simulink model "ComfortMdRStEnCtrl"  (R2018b)
settings: Solver=FixedStepDiscrete  StartTime=0.0  StopTime=10.0  FixedStep=0.01  RelTol=1e-3
undefined symbols (not defined in the file or in its folder): data, KeSMSw4SSecRwLtStLgrstOtwdInwdClosePos1_Val, KeSMSw4SSecRwLtStLgrstUpwdDnwdClosePos1_Val, KeSMSw4SSecRwLtStLgrstUpwdDnwdClosePos2_Val, KeSMSw4SSecRwRtStLgrstUpwdDnwdOpenPos1_Val, SecRwRtStBkRclnEn_Clear, SecRwRtStBkRclnEn_Set, SecRwRtStLgrstInwdOtwdEn_Clear, SecRwRtStLgrstInwdOtwdEn_Set, SecRwRtStLgrstUpwdDnwdEn_Clear, SecRwRtStLgrstUpwdDnwdEn_Set, ZeroREn_Clear, ZeroREn_Set
libraries: simulink x1
settings Model: Creator=sn2xws  LastModifiedBy=sn2xws
settings Model: ModifiedHistory=|
  | 2024.6.19 V1.1.0 模式流程V1.6
  | 2025.4.18 V1.10.0 腿托收流程中标定使用错误问题修复
settings DataIOCC: SaveFormat=StructureWithTime
settings OptimizationCC: DefaultParameterBehavior=Inlined  EnhancedBackFolding=on  PassReuseOutputArgsAs=Individual arguments  ZeroExternalMemoryAtStartup=off  ZeroInternalMemoryAtStartup=off  OptimizeBlockOrder=speed  DifferentSizesBufferReuse=on  OptimizationCustomize=off
settings DebuggingCC: ParameterTunabilityLossMsg=error
settings SFSimCC: MATLABDynamicMemAlloc=off
settings RTWCC: SystemTargetFile=autosar.tlc  GenCodeOnly=on  TemplateMakefile=ert_default_tmf  Description=AUTOSAR  GenerateReport=on  IncludeHyperlinkInReport=on  LaunchReport=on  GenerateTraceInfo=on  GenerateTraceReport=on  GenerateTraceReportSl=on  GenerateTraceReportSf=on  GenerateTraceReportEml=on
settings CodeAppCC: ForceParamTrailComments=on  IgnoreCustomStorageClasses=off  OperatorAnnotations=on  SimulinkDataObjDesc=on  SFDataObjDesc=on  InsertBlockDesc=on
settings STFCustomTargetCC: TargetLangStandard=C99 (ISO)  MultiwordLength=256  ParMdlRefBuildCompliant=on  CompOptLevelCompliant=on  IncludeMdlTerminateFcn=off  CombineOutputUpdateFcns=on  SuppressErrorStatus=on  ERTCustomFileBanners=on  SupportNonFinite=off  SupportComplex=off  SupportContinuousTime=off  SupportNonInlinedSFcns=off  RemoveResetFunc=on  MATLABClassNameForMDSCustomization=Simulink.SoftwareTarget.ERTCustomization  AutosarCompliant=on  UseToolchainInfoCompliant=on  LookupTableObjectStructAxisOrder=2,1,3,4,...  LUTObjectStructOrderEvenSpacing=Size,Table,Breakpoints  SystemTargetFile=autosar.tlc
settings ERTTargetCC: TargetLangStandard=C99 (ISO)  ConcurrentExecutionCompliant=off  IncludeMdlTerminateFcn=off  SuppressErrorStatus=on  SupportNonFinite=off  SupportComplex=off  ModelStepFunctionPrototypeControlCompliant=off  CPPClassGenCompliant=off  AutosarCompliant=on  LookupTableObjectStructAxisOrder=2,1,3,4,...  LUTObjectStructOrderEvenSpacing=Size,Table,Breakpoints  InlinedParameterPlacement=NonHierarchical  ERTCustomFileTemplate=example_file_process.tlc  ERTFilePackagingFormat=Compact

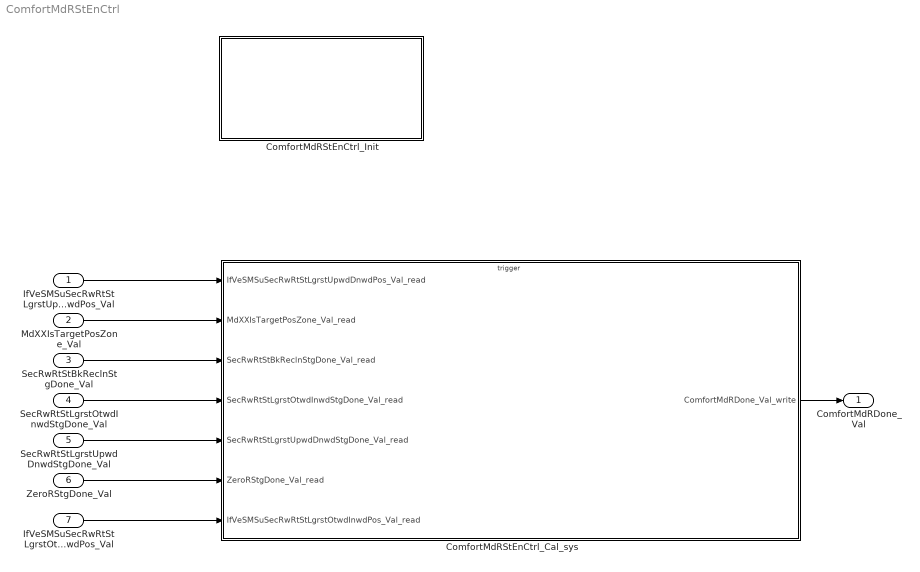
== system ComfortMdRStEnCtrl ==
  IfVeSMSuSecRwRtStLgrstUpwdDnwdPos_Val : Inport  OutDataTypeStr=uint16  PortDimensions=1
  MdXXIsTargetPosZone_Val : Inport  Port=2  OutDataTypeStr=uint32  PortDimensions=1
  SecRwRtStBkReclnStgDone_Val : Inport  Port=3  OutDataTypeStr=boolean  PortDimensions=1
  SecRwRtStLgrstOtwdInwdStgDone_Val : Inport  Port=4  OutDataTypeStr=boolean  PortDimensions=1
  SecRwRtStLgrstUpwdDnwdStgDone_Val : Inport  Port=5  OutDataTypeStr=boolean  PortDimensions=1
  ZeroRStgDone_Val : Inport  Port=6  OutDataTypeStr=boolean  PortDimensions=1
  IfVeSMSuSecRwRtStLgrstOtwdInwdPos_Val : Inport  Port=7  OutDataTypeStr=uint16  PortDimensions=1
  ComfortMdRStEnCtrl_Cal_sys : Subsystem
  ComfortMdRStEnCtrl_Init : Subsystem
  ComfortMdRDone_Val : Outport  OutDataTypeStr=uint8  PortDimensions=1
  wires:
  IfVeSMSuSecRwRtStLgrstUpwdDnwdPos_Val/1 -> ComfortMdRStEnCtrl_Cal_sys/1(IfVeSMSuSecRwRtStLgrstUpwdDnwdPos_Val_read)
  MdXXIsTargetPosZone_Val/1 -> ComfortMdRStEnCtrl_Cal_sys/2(MdXXIsTargetPosZone_Val_read)
  SecRwRtStBkReclnStgDone_Val/1 -> ComfortMdRStEnCtrl_Cal_sys/3(SecRwRtStBkReclnStgDone_Val_read)
  SecRwRtStLgrstOtwdInwdStgDone_Val/1 -> ComfortMdRStEnCtrl_Cal_sys/4(SecRwRtStLgrstOtwdInwdStgDone_Val_read)
  SecRwRtStLgrstUpwdDnwdStgDone_Val/1 -> ComfortMdRStEnCtrl_Cal_sys/5(SecRwRtStLgrstUpwdDnwdStgDone_Val_read)
  ZeroRStgDone_Val/1 -> ComfortMdRStEnCtrl_Cal_sys/6(ZeroRStgDone_Val_read)
  ComfortMdRStEnCtrl_Cal_sys/1(ComfortMdRDone_Val_write) -> ComfortMdRDone_Val/1
  IfVeSMSuSecRwRtStLgrstOtwdInwdPos_Val/1 -> ComfortMdRStEnCtrl_Cal_sys/7(IfVeSMSuSecRwRtStLgrstOtwdInwdPos_Val_read)

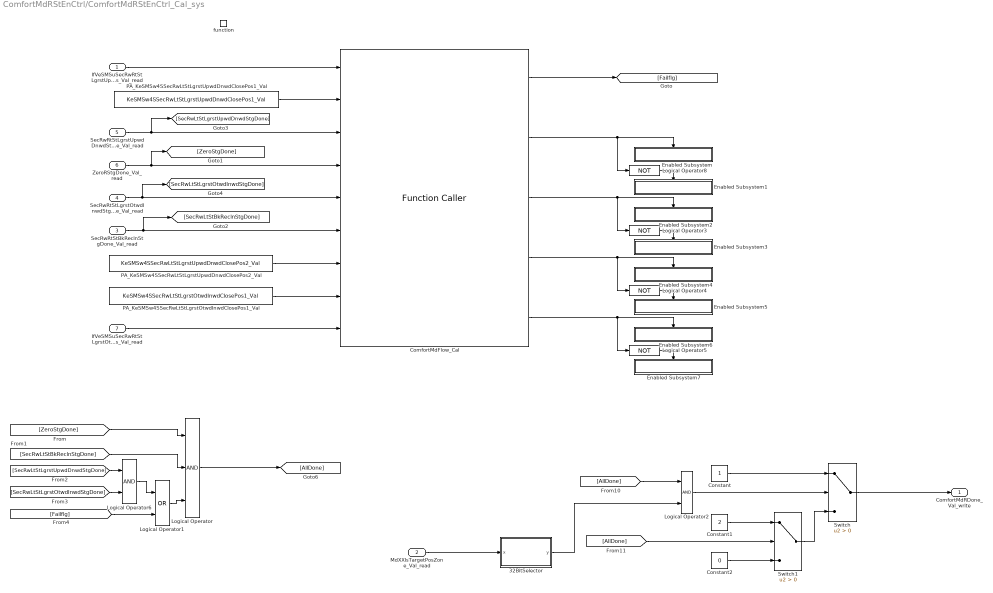
== system ComfortMdRStEnCtrl/ComfortMdRStEnCtrl_Cal_sys ==
  IfVeSMSuSecRwRtStLgrstUpwdDnwdPos_Val_read : Inport
  MdXXIsTargetPosZone_Val_read : Inport  Port=2
  SecRwRtStBkReclnStgDone_Val_read : Inport  Port=3
  SecRwRtStLgrstOtwdInwdStgDone_Val_read : Inport  Port=4
  SecRwRtStLgrstUpwdDnwdStgDone_Val_read : Inport  Port=5
  ZeroRStgDone_Val_read : Inport  Port=6
  IfVeSMSuSecRwRtStLgrstOtwdInwdPos_Val_read : Inport  Port=7
  function : TriggerPort  TriggerType=function-call  IsSimulinkFunction=on  FunctionName=ComfortMdRStEnCtrl_Cal  VariantControl=(inherit)
  32BitSelector : Subsystem  mask(32 Bit Selector){BitNum=12}
      mask prompts: BitNum "Select Bit Number"
      mask help: Allows selection of a particular bit (0-31) out of a packed word up to 32 bits long. Output will be true if the bit number selected via the mask parameter is equal to one.
      mask TypeOptions BitNum: 0 | 1 | 2 | 3 | 4 | 5 | 6 | 7 | 8 | 9 | 10 | 11 | 12 | 13 | 14 | 15 | 16 | 17 | 18 | 19 | 20 | 21 | 22 | 23 | 24 | 25 | 26 | 27 | 28 | 29 | 30 | 31
      mask Display:
      | text(0.5, 0.8,'BIT','horizontalAlignment','center')
      | text(0.5, 0.5,'SELECTOR','horizontalAlignment','center')
      | text(0.5, 0.2,['-- Bit ',char(get_param(gcb,'BitNum')),' --'],'horizontalAlignment','center')
  ComfortMdFlow_Cal : FunctionCaller  FunctionPrototype=[Failflg,LgrstInwdOtwdEn,LgrstUpwdDnwdEn,ZeroEn,BkReclnEn] = ComfortMdFlow_Cal(LgrstUpwdDnwdPos,LgrstUpwdDnwdClosePos1,LgrstUpwdStgDone,ZeroStgDone,LgrstInwdStgDone,BkReclnStgDone,LgrstUpwdDnwdClosePos2,LgrstInwdOtwdClosePos1,LgrstInwdOtwdPos)  InputArgumentSpecifications=uint16(1), uint16(1), boolean(true), boolean(true), boolean(true), boolean(true), uint16(1), uint16(1), uint16(1)  OutputArgumentSpecifications=boolean(true), boolean(true), boolean(true), boolean(true), boolean(true)
  Constant : Constant  OutDataTypeStr=uint8
  Constant1 : Constant  Value=2  OutDataTypeStr=uint8
  Constant2 : Constant  Value=0  OutDataTypeStr=uint8
  Enabled Subsystem : Subsystem  TreatAsAtomicUnit=on
  Enabled Subsystem1 : Subsystem  TreatAsAtomicUnit=on
  Enabled Subsystem2 : Subsystem  TreatAsAtomicUnit=on
  Enabled Subsystem3 : Subsystem  TreatAsAtomicUnit=on
  Enabled Subsystem4 : Subsystem  TreatAsAtomicUnit=on
  Enabled Subsystem5 : Subsystem  TreatAsAtomicUnit=on
  Enabled Subsystem6 : Subsystem  TreatAsAtomicUnit=on
  Enabled Subsystem7 : Subsystem  TreatAsAtomicUnit=on
  Logical Operator : Logic  Inputs=3  AllPortsSameDT=off  OutDataTypeStr=boolean
  Logical Operator1 : Logic  Operator=OR  AllPortsSameDT=off  OutDataTypeStr=boolean
  Logical Operator2 : Logic  AllPortsSameDT=off  OutDataTypeStr=boolean
  Logical Operator{3..5,8} (4 alike) : Logic  Operator=NOT  AllPortsSameDT=off  OutDataTypeStr=boolean
  Logical Operator6 : Logic  AllPortsSameDT=off  OutDataTypeStr=boolean
  PA_KeSMSw4SSecRwLtStLgrstOtwdInwdClosePos1_Val : Constant  Value=KeSMSw4SSecRwLtStLgrstOtwdInwdClosePos1_Val
  PA_KeSMSw4SSecRwLtStLgrstUpwdDnwdClosePos1_Val : Constant  Value=KeSMSw4SSecRwLtStLgrstUpwdDnwdClosePos1_Val
  PA_KeSMSw4SSecRwLtStLgrstUpwdDnwdClosePos2_Val : Constant  Value=KeSMSw4SSecRwLtStLgrstUpwdDnwdClosePos2_Val
  Switch : Switch  Criteria=u2 > Threshold
  Switch1 : Switch  Criteria=u2 > Threshold
  ComfortMdRDone_Val_write : Outport
      settings: EnsureOutportIsVirtual=on
  wires:
  IfVeSMSuSecRwRtStLgrstUpwdDnwdPos_Val_read/1 -> ComfortMdFlow_Cal/1
  SecRwRtStLgrstUpwdDnwdStgDone_Val_read/1 -> [SecRwLtStLgrstUpwdDnwdStgDone], ComfortMdFlow_Cal/3
  ZeroRStgDone_Val_read/1 -> [ZeroStgDone], ComfortMdFlow_Cal/4
  SecRwRtStLgrstOtwdInwdStgDone_Val_read/1 -> [SecRwLtStLgrstOtwdInwdStgDone], ComfortMdFlow_Cal/5
  SecRwRtStBkReclnStgDone_Val_read/1 -> [SecRwLtStBkReclnStgDone], ComfortMdFlow_Cal/6
  [SecRwLtStBkReclnStgDone] -> Logical Operator/2
  Logical Operator/1 -> [AllDone]
  [ZeroStgDone] -> Logical Operator/1
  Logical Operator1/1 -> Logical Operator/3
  32BitSelector/1(y) -> Logical Operator2/2
  Constant2/1 -> Switch1/3
  Switch/1 -> ComfortMdRDone_Val_write/1
  MdXXIsTargetPosZone_Val_read/1 -> 32BitSelector/1(x)
  Constant/1 -> Switch/1
  Switch1/1 -> Switch/3
  [AllDone] -> Switch1/2
  Logical Operator2/1 -> Switch/2
  [AllDone] -> Logical Operator2/1
  Constant1/1 -> Switch1/1
  ComfortMdFlow_Cal/1 -> [Failflg]
  Logical Operator8/1 -> Enabled Subsystem1/Enable
  ComfortMdFlow_Cal/2 -> Logical Operator8/1, Enabled Subsystem/Enable
  ComfortMdFlow_Cal/3 -> Enabled Subsystem2/Enable, Logical Operator3/1
  Logical Operator3/1 -> Enabled Subsystem3/Enable
  Logical Operator4/1 -> Enabled Subsystem5/Enable
  ComfortMdFlow_Cal/4 -> Logical Operator4/1, Enabled Subsystem4/Enable
  ComfortMdFlow_Cal/5 -> Enabled Subsystem6/Enable, Logical Operator5/1
  Logical Operator5/1 -> Enabled Subsystem7/Enable
  [Failflg] -> Logical Operator1/2
  PA_KeSMSw4SSecRwLtStLgrstUpwdDnwdClosePos2_Val/1 -> ComfortMdFlow_Cal/7
  IfVeSMSuSecRwRtStLgrstOtwdInwdPos_Val_read/1 -> ComfortMdFlow_Cal/9
  [SecRwLtStLgrstOtwdInwdStgDone] -> Logical Operator6/2
  [SecRwLtStLgrstUpwdDnwdStgDone] -> Logical Operator6/1
  Logical Operator6/1 -> Logical Operator1/1
  PA_KeSMSw4SSecRwLtStLgrstUpwdDnwdClosePos1_Val/1 -> ComfortMdFlow_Cal/2
  PA_KeSMSw4SSecRwLtStLgrstOtwdInwdClosePos1_Val/1 -> ComfortMdFlow_Cal/8

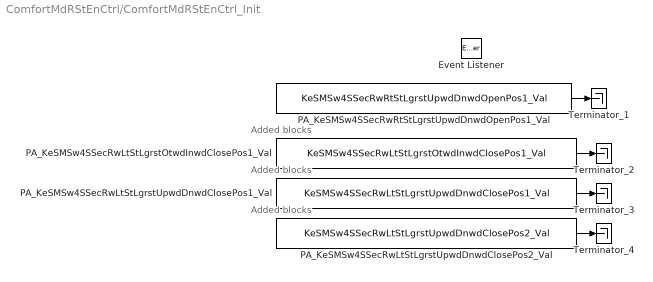
== system ComfortMdRStEnCtrl/ComfortMdRStEnCtrl_Init ==
  note: Added blocks
  note: Added blocks
  note: Added blocks
  Event Listener : EventListener  EventName=reset
  PA_KeSMSw4SSecRwLtStLgrstOtwdInwdClosePos1_Val : Constant  Value=KeSMSw4SSecRwLtStLgrstOtwdInwdClosePos1_Val
  PA_KeSMSw4SSecRwLtStLgrstUpwdDnwdClosePos1_Val : Constant  Value=KeSMSw4SSecRwLtStLgrstUpwdDnwdClosePos1_Val
  PA_KeSMSw4SSecRwLtStLgrstUpwdDnwdClosePos2_Val : Constant  Value=KeSMSw4SSecRwLtStLgrstUpwdDnwdClosePos2_Val
  PA_KeSMSw4SSecRwRtStLgrstUpwdDnwdOpenPos1_Val : Constant  Value=KeSMSw4SSecRwRtStLgrstUpwdDnwdOpenPos1_Val
  Terminator_{1..4} (4 alike) : Terminator
  wires:
  PA_KeSMSw4SSecRwRtStLgrstUpwdDnwdOpenPos1_Val/1 -> Terminator_1/1
  PA_KeSMSw4SSecRwLtStLgrstOtwdInwdClosePos1_Val/1 -> Terminator_2/1
  PA_KeSMSw4SSecRwLtStLgrstUpwdDnwdClosePos1_Val/1 -> Terminator_3/1
  PA_KeSMSw4SSecRwLtStLgrstUpwdDnwdClosePos2_Val/1 -> Terminator_4/1

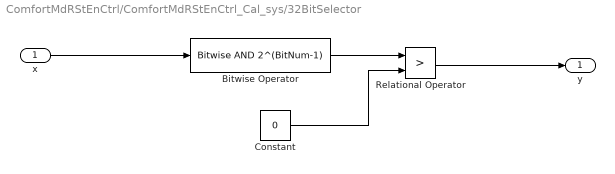
== system ComfortMdRStEnCtrl/ComfortMdRStEnCtrl_Cal_sys/32BitSelector ==
  x : Inport
  Bitwise Operator : simulink/Logic and Bit Operations/Bitwise Operator  logicop=AND  UseBitMask=on  BitMask=2^(BitNum-1)  BitMaskRealWorld=Stored Integer
  Constant : Constant  Value=0  OutDataTypeStr=uint32
  Relational Operator : RelationalOperator  Operator=>  OutDataTypeStr=boolean  RndMeth=Simplest
  y : Outport
  wires:
  Relational Operator/1 -> y/1
  Constant/1 -> Relational Operator/2
  x/1 -> Bitwise Operator/1
  Bitwise Operator/1 -> Relational Operator/1

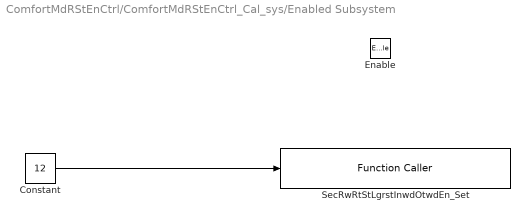
== system ComfortMdRStEnCtrl/ComfortMdRStEnCtrl_Cal_sys/Enabled Subsystem ==
  Enable : EnablePort
  Constant : Constant  Value=12  OutDataTypeStr=uint8
  SecRwRtStLgrstInwdOtwdEn_Set : FunctionCaller  FunctionPrototype=SecRwRtStLgrstInwdOtwdEn_Set(data)  InputArgumentSpecifications=uint8(1)
  wires:
  Constant/1 -> SecRwRtStLgrstInwdOtwdEn_Set/1

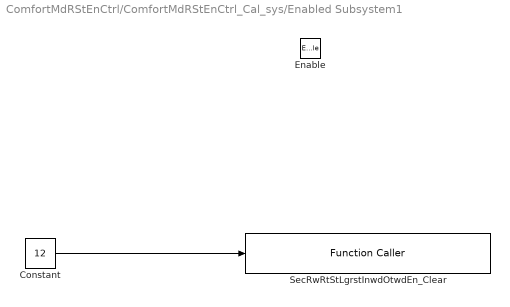
== system ComfortMdRStEnCtrl/ComfortMdRStEnCtrl_Cal_sys/Enabled Subsystem1 ==
  Enable : EnablePort
  Constant : Constant  Value=12  OutDataTypeStr=uint8
  SecRwRtStLgrstInwdOtwdEn_Clear : FunctionCaller  FunctionPrototype=SecRwRtStLgrstInwdOtwdEn_Clear(data)  InputArgumentSpecifications=uint8(1)
  wires:
  Constant/1 -> SecRwRtStLgrstInwdOtwdEn_Clear/1

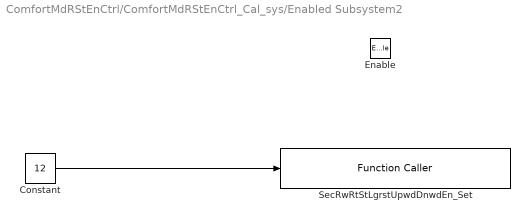
== system ComfortMdRStEnCtrl/ComfortMdRStEnCtrl_Cal_sys/Enabled Subsystem2 ==
  Enable : EnablePort
  Constant : Constant  Value=12  OutDataTypeStr=uint8
  SecRwRtStLgrstUpwdDnwdEn_Set : FunctionCaller  FunctionPrototype=SecRwRtStLgrstUpwdDnwdEn_Set(data)  InputArgumentSpecifications=uint8(1)
  wires:
  Constant/1 -> SecRwRtStLgrstUpwdDnwdEn_Set/1

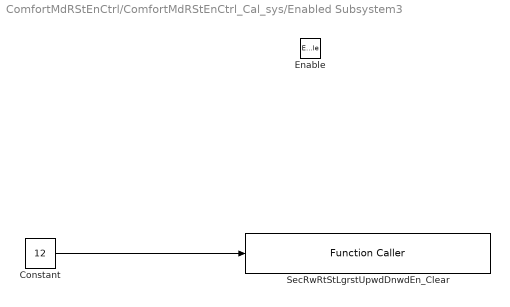
== system ComfortMdRStEnCtrl/ComfortMdRStEnCtrl_Cal_sys/Enabled Subsystem3 ==
  Enable : EnablePort
  Constant : Constant  Value=12  OutDataTypeStr=uint8
  SecRwRtStLgrstUpwdDnwdEn_Clear : FunctionCaller  FunctionPrototype=SecRwRtStLgrstUpwdDnwdEn_Clear(data)  InputArgumentSpecifications=uint8(1)
  wires:
  Constant/1 -> SecRwRtStLgrstUpwdDnwdEn_Clear/1

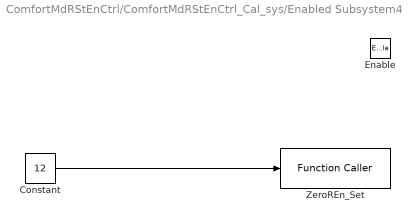
== system ComfortMdRStEnCtrl/ComfortMdRStEnCtrl_Cal_sys/Enabled Subsystem4 ==
  Enable : EnablePort
  Constant : Constant  Value=12  OutDataTypeStr=uint8
  ZeroREn_Set : FunctionCaller  FunctionPrototype=ZeroREn_Set(data)  InputArgumentSpecifications=uint8(1)
  wires:
  Constant/1 -> ZeroREn_Set/1

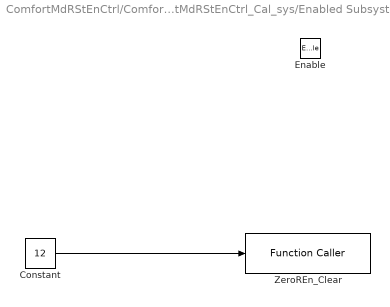
== system ComfortMdRStEnCtrl/ComfortMdRStEnCtrl_Cal_sys/Enabled Subsystem5 ==
  Enable : EnablePort
  Constant : Constant  Value=12  OutDataTypeStr=uint8
  ZeroREn_Clear : FunctionCaller  FunctionPrototype=ZeroREn_Clear(data)  InputArgumentSpecifications=uint8(1)
  wires:
  Constant/1 -> ZeroREn_Clear/1

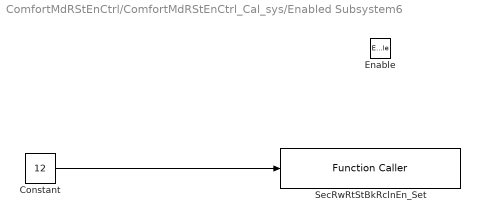
== system ComfortMdRStEnCtrl/ComfortMdRStEnCtrl_Cal_sys/Enabled Subsystem6 ==
  Enable : EnablePort
  Constant : Constant  Value=12  OutDataTypeStr=uint8
  SecRwRtStBkRclnEn_Set : FunctionCaller  FunctionPrototype=SecRwRtStBkRclnEn_Set(data)  InputArgumentSpecifications=uint8(1)
  wires:
  Constant/1 -> SecRwRtStBkRclnEn_Set/1

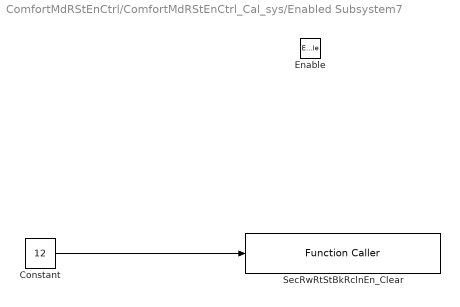
== system ComfortMdRStEnCtrl/ComfortMdRStEnCtrl_Cal_sys/Enabled Subsystem7 ==
  Enable : EnablePort
  Constant : Constant  Value=12  OutDataTypeStr=uint8
  SecRwRtStBkRclnEn_Clear : FunctionCaller  FunctionPrototype=SecRwRtStBkRclnEn_Clear(data)  InputArgumentSpecifications=uint8(1)
  wires:
  Constant/1 -> SecRwRtStBkRclnEn_Clear/1
